simulink model "Shay_Problem_16_10"  (R2018b)
settings: Solver=VariableStepAuto  StartTime=0.0  StopTime=10.0  RelTol=1e-3
settings Model: Creator=labstudent  LastModifiedBy=labstudent

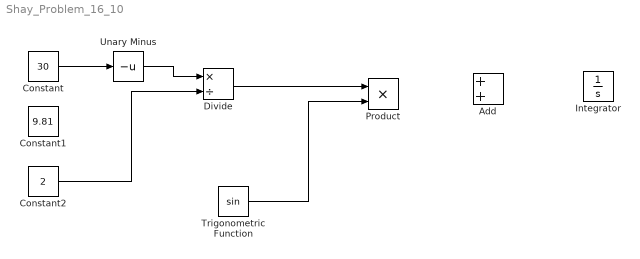
== system Shay_Problem_16_10 ==
  Add : Sum
  Constant : Constant  Value=30
  Constant1 : Constant  Value=9.81
  Constant2 : Constant  Value=2
  Divide : Product  Inputs=*/
  Integrator : Integrator
  Product : Product
  Trigonometric Function : Trigonometry
  Unary Minus : UnaryMinus
  wires:
  Constant/1 -> Unary Minus/1
  Unary Minus/1 -> Divide/1
  Constant2/1 -> Divide/2
  Divide/1 -> Product/1
  Trigonometric Function/1 -> Product/2
